simulink model "TractionCtrl"  (R2020a)
settings: Solver=VariableStepAuto  StartTime=0.0  StopTime=10.0  RelTol=1e-3
model workspace (MAT data in the model file):
  aimSlipLookupTable = [25  0  0  0  0  0  0  0  0  0  0  0; 25  0  0  0  0  0  0  0  0  0  0  0; 25  23  23  0  0  0  0  0  0  0  0  0; 25  23  23  0  0  0  0  0  0  0  0  0; 25  0  0  18  25  25  25  25  25  0  0  0; 25  0  0  18  25  25  20  25  25  0  0  0; 25  0  0  0  0  0  0  0  0  0  0  0; 25  0  0  0  0  0  0  0  0  0  0  0; 25  0  0  0  0  0  0  0  0  0  0  0; 25  0  0  0  0  0  0  0  0  0  0  0; 25  25  25  25  25  25  25  25  25  25  10  10]
libraries: simulink x1
settings Model: Creator=44689  LastModifiedBy=44689

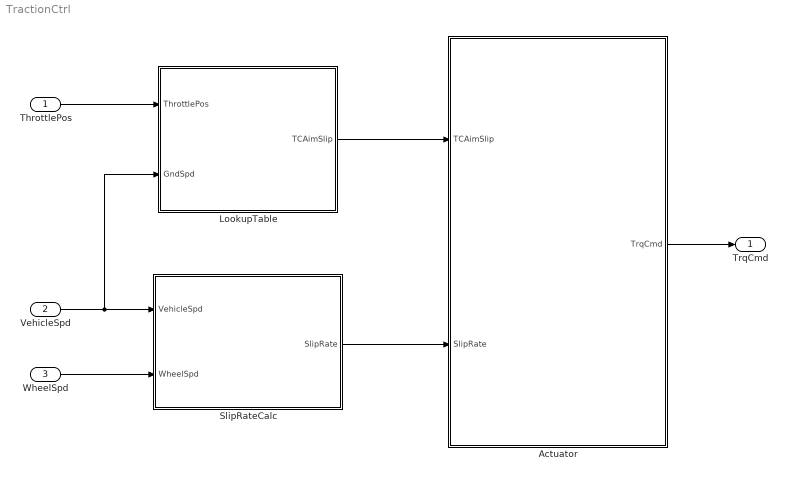
== system TractionCtrl ==
  ThrottlePos : Inport
  VehicleSpd : Inport  Port=2
  WheelSpd : Inport  Port=3
  Actuator : Subsystem
  LookupTable : Subsystem
  SlipRateCalc : Subsystem
  TrqCmd : Outport
  wires:
  ThrottlePos/1 -> LookupTable/1(ThrottlePos)
  VehicleSpd/1 -> LookupTable/2(GndSpd), SlipRateCalc/1(VehicleSpd)
  WheelSpd/1 -> SlipRateCalc/2(WheelSpd)
  LookupTable/1(TCAimSlip) -> Actuator/1(TCAimSlip)
  SlipRateCalc/1(SlipRate) -> Actuator/2(SlipRate)
  Actuator/1(TrqCmd) -> TrqCmd/1

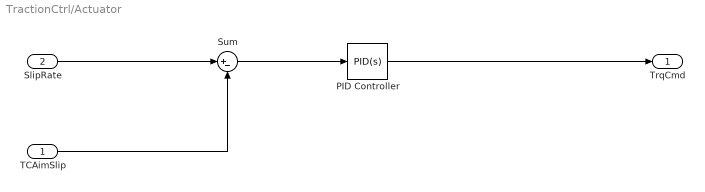
== system TractionCtrl/Actuator ==
  TCAimSlip : Inport
  SlipRate : Inport  Port=2
  PID Controller : simulink/Continuous/PID Controller  Controller=PID  Form=Parallel  TimeDomain=Continuous-time  UseExternalTs=off  SampleTime=-1  IntegratorMethod=Forward Euler  FilterMethod=Forward Euler  ControllerParametersSource=internal  P=1  I=1  D=0  UseFilter=on  N=100  TunerSelectOption=Transfer Function Based (PID Tuner App)  InitialConditionSource=internal  InitialConditionForIntegrator=0  InitialConditionForFilter=0  DifferentiatorICPrevScaledInput=0  ExternalReset=none  TrackingMode=off  Kt=1  LimitOutput=off  UpperSaturationLimit=inf  LowerSaturationLimit=-inf  LinearizeAsGain=on  AntiWindupMode=none  Kb=1  POutMin=[]  POutMax=[]  IOutMin=[]  IOutMax=[]  DOutMin=[]  DOutMax=[]  NOutMin=[]  NOutMax=[]  SumOutMin=[]  SumOutMax=[]  SaturationOutMin=[]  SaturationOutMax=[]  PParamMin=[]  PParamMax=[]  IParamMin=[]  IParamMax=[]  DParamMin=[]  DParamMax=[]  NParamMin=[]  NParamMax=[]  KbParamMin=[]  KbParamMax=[]  KtParamMin=[]  KtParamMax=[]  KbOutMin=[]  KbOutMax=[]  KtOutMin=[]  KtOutMax=[]  IntegratorOutMin=[]  IntegratorOutMax=[]  FilterOutMin=[]  FilterOutMax=[]  SumI1OutMin=[]  SumI1OutMax=[]  SumI2OutMin=[]  SumI2OutMax=[]  SumI3OutMin=[]  SumI3OutMax=[]  SumI4OutMin=[]  SumI4OutMax=[]  SumDOutMin=[]  SumDOutMax=[]  DifferentiatorOutMin=[]  DifferentiatorOutMax=[]  FilterDiffOutCoefMin=[]  FilterDiffOutCoefMax=[]  ReciprocalOutMin=[]  ReciprocalOutMax=[]  SumDenOutMin=[]  SumDenOutMax=[]  SumNumOutMin=[]  SumNumOutMax=[]  DivideOutMin=[]  DivideOutMax=[]  UdiffTsProdOutMin=[]  UdiffTsProdOutMax=[]  NTsProdOutMin=[]  NTsProdOutMax=[]  UintegralTsProdOutMin=[]  UintegralTsProdOutMax=[]  UngainTsProdOutMin=[]  UngainTsProdOutMax=[]  IntegratorContinuousStateAttributes=''  IntegratorStateMustResolveToSignalObject=off  IntegratorRTWStateStorageClass=Auto  FilterContinuousStateAttributes=''  FilterStateMustResolveToSignalObject=off  FilterRTWStateStorageClass=Auto  ParallelPVariant=InternalParameters  IdealPVariant=Disabled  IVariant=InternalParameters  DVariant=InternalParameters  IntegratorVariant=Continuous  SatVariant=Disabled  AWVariant=Passthrough  PCopyVariant=Disabled  TRVariant=Disabled  FdbkBlocksVariant=Forward  IdealPFdbkVariant=Disabled  SatFdbkVariant=Disabled  DerivativeFilterVariant=ContFilter  NVariant=InternalParameters  NCopyVariant=Disabled  FilterICVariant=InternalICsFilter  IntegratorICVariant=InternalICs  ExternalResetVariant=Disabled  TRSumVariant=Passthrough  SumFdbkVariant=Disabled  SumVariant=Sum_PID  TsampFilterVariant=InternalTs  TsampNgainVariant=Passthrough  TsampIntegralVariant=Passthrough
  Sum : Sum  Inputs=|+-
  TrqCmd : Outport
  wires:
  SlipRate/1 -> Sum/1
  Sum/1 -> PID Controller/1
  PID Controller/1 -> TrqCmd/1
  TCAimSlip/1 -> Sum/2

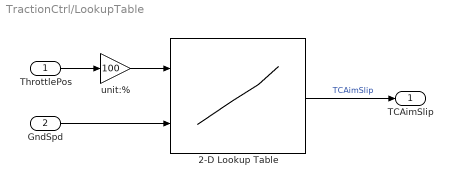
== system TractionCtrl/LookupTable ==
  ThrottlePos : Inport
  GndSpd : Inport  Port=2
  2-D Lookup Table : Lookup_n-D  BreakpointsForDimension1=[0 5 8 10 20 30 40 50 60 70 100]  BreakpointsForDimension2=[0 10 20 30 40 45 50 55 60 70 90 100]  Table=aimSlipLookupTable  InternalRulePriority=Speed  RndMeth=Simplest  InputSameDT=on
  unit:% : Gain  Gain=100
  TCAimSlip : Outport
  wires:
  ThrottlePos/1 -> unit:%/1
  GndSpd/1 -> 2-D Lookup Table/2
  2-D Lookup Table/1 -> TCAimSlip/1  "TCAimSlip"
  unit:%/1 -> 2-D Lookup Table/1

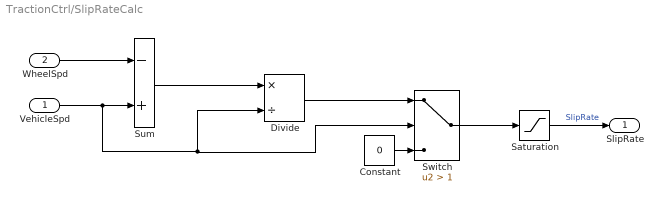
== system TractionCtrl/SlipRateCalc ==
  VehicleSpd : Inport
  WheelSpd : Inport  Port=2
  Constant : Constant  Value=0
  Divide : Product  Inputs=*/
  Saturation : Saturate  UpperLimit=1  LowerLimit=0
  Sum : Sum  Inputs=-+
  Switch : Switch  Criteria=u2 > Threshold  Threshold=1
  SlipRate : Outport
  wires:
  Divide/1 -> Switch/1
  Constant/1 -> Switch/3
  Saturation/1 -> SlipRate/1  "SlipRate"
  Switch/1 -> Saturation/1
  WheelSpd/1 -> Sum/1
  Sum/1 -> Divide/1
  VehicleSpd/1 -> Switch/2, Divide/2, Sum/2
